simulink model "noise_model_simulink_spectrum_sb"  (R2019b)
settings: Solver=VariableStepAuto  StartTime=0.0  StopTime=60  RelTol=1e-3
libraries: dspsrcs4 x2
settings Model: Creator=Carolina  LastModifiedBy=sbuccelli
settings SFSimCC: CustomCodeUndefinedFunction=UseInterfaceOnly

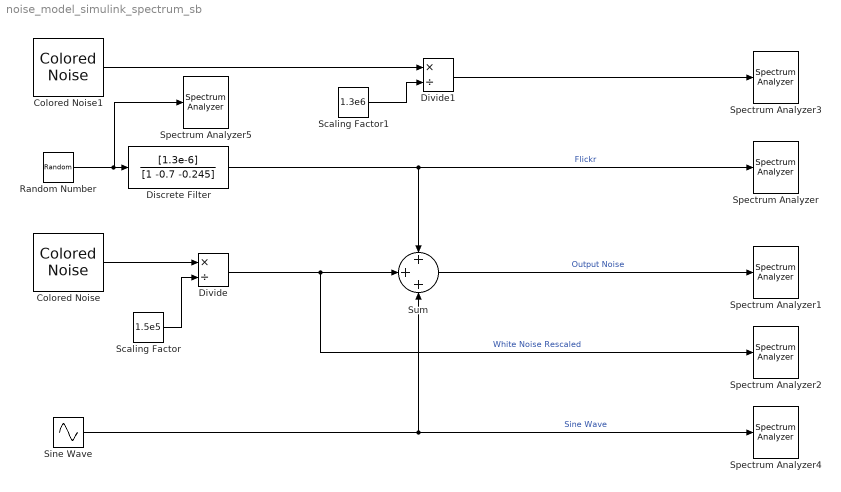
== system noise_model_simulink_spectrum_sb ==
  Colored Noise : dspsrcs4/Colored Noise  Color=white  InverseFrequencyPower=1  BoundedOutput=off  NumChannels=1  OutputDataType=double  SamplesPerFrame=1  SampleTime=1/24414  RandomStream=mt19937ar with seed  Seed=67  SimulateUsing=Interpreted execution
      settings: SourceProductName=DSP System Toolbox  SourceProductBaseCode=DS
  Colored Noise1 : dspsrcs4/Colored Noise  Color=custom  InverseFrequencyPower=1.4  BoundedOutput=off  NumChannels=1  OutputDataType=double  SamplesPerFrame=1  SampleTime=1/24414  RandomStream=mt19937ar with seed  Seed=67  SimulateUsing=Interpreted execution
      settings: SourceProductName=DSP System Toolbox  SourceProductBaseCode=DS
  Discrete Filter : DiscreteFilter  Numerator=[1.3e-6]  Denominator=[1 -0.7 -0.245]
  Divide : Product  Inputs=*/
  Divide1 : Product  Inputs=*/
  Random Number : RandomNumber  Seed=67  SampleTime=1/24414
  Scaling Factor : Constant  Value=1.5e5
  Scaling Factor1 : Constant  Value=1.3e6
  Sine Wave : Sin  Amplitude=0.6e-6  Frequency=314.16  SampleTime=1/24414
  Spectrum Analyzer{,1..5} (6 alike) : SpectrumAnalyzer
  Sum : Sum  Inputs=+++
  wires:
  Sine Wave/1 -> Sum/3, Spectrum Analyzer4/1  "Sine Wave"
  Sum/1 -> Spectrum Analyzer1/1  "Output Noise"
  Random Number/1 -> Spectrum Analyzer5/1, Discrete Filter/1
  Colored Noise/1 -> Divide/1
  Divide/1 -> Spectrum Analyzer2/1, Sum/2  "White Noise Rescaled"
  Scaling Factor/1 -> Divide/2
  Discrete Filter/1 -> Sum/1, Spectrum Analyzer/1  "Flickr"
  Scaling Factor1/1 -> Divide1/2
  Colored Noise1/1 -> Divide1/1
  Divide1/1 -> Spectrum Analyzer3/1
